simulink model "Galvo_sys_Ccont_Pcont_cc_nosub_bandwidth_v69_linmod"  (R2015a)
settings: Solver=ode45  StartTime=0.0  StopTime=10.0  RelTol=1e-3
undefined symbols (not defined in the file or in its folder): ccKp, dPosMax, JR, KEL, KEMF, KFR, KSH, KTB, Lc, RL, Rsh
libraries: simulink x2
settings Model: DataDictionary=modelDesignData_Galvo_sys_Ccont_Pcont.sldd  Creator=mainster  LastModifiedBy=mainster
settings DebuggingCC: InitInArrayFormatMsg=none

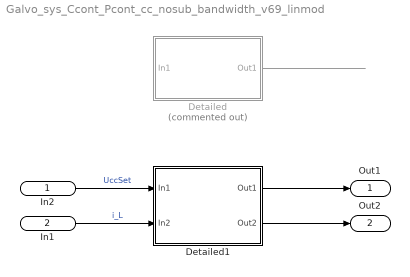
== system Galvo_sys_Ccont_Pcont_cc_nosub_bandwidth_v69_linmod ==
  In2 : Inport
  In1 : Inport  Port=2
  Detailed : Subsystem  Commented=on
  Detailed1 : Subsystem
  Out1 : Outport
  Out2 : Outport  Port=2
  wires:
  ? -> Detailed/1(In1)  "UccSet"
  Detailed/1(Out1) -> ?
  In2/1 -> Detailed1/1(In1)  "UccSet"
  Detailed1/1(Out1) -> Out1/1
  In1/1 -> Detailed1/2(In2)  "i_L"
  Detailed1/2(Out2) -> Out2/1

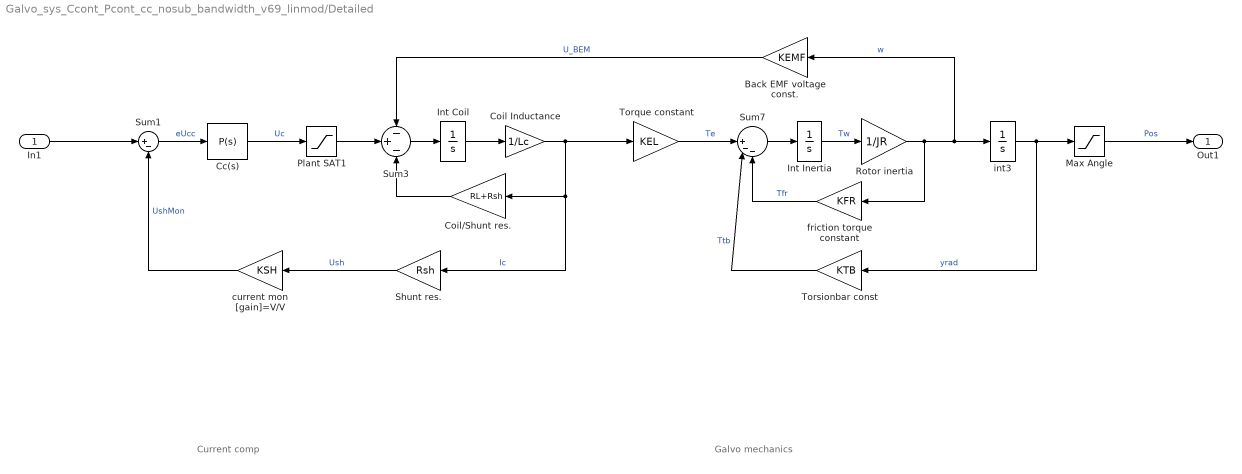
== system Galvo_sys_Ccont_Pcont_cc_nosub_bandwidth_v69_linmod/Detailed ==
  note: Galvo mechanics
  note: Current comp
  In1 : Inport
  Back EMF voltage const. : Gain  RequirementInfo={} %GIDa_1b5a4587_d3eb_4817_81be_45424a09f54c  Gain=KEMF
  Cc(s) : simulink/Continuous/PID Controller  Controller=P  TimeDomain=Continuous-time  SampleTime=-1  IntegratorMethod=Forward Euler  FilterMethod=Forward Euler  Form=Ideal  UseFilter=on  ControllerParametersSource=internal  P=ccKp  I=79241.5509357268  D=0  N=100  InitialConditionSource=internal  InitialConditionForIntegrator=0  InitialConditionForFilter=0  ExternalReset=none  LimitOutput=off  UpperSaturationLimit=inf  LowerSaturationLimit=-inf  LinearizeAsGain=on  AntiWindupMode=none  Kb=1  TrackingMode=off  Kt=1  PParamMin=[]  PParamMax=[]  IParamMin=[]  IParamMax=[]  DParamMin=[]  DParamMax=[]  NParamMin=[]  NParamMax=[]  KbParamMin=[]  KbParamMax=[]  KtParamMin=[]  KtParamMax=[]  POutMin=[]  POutMax=[]  IOutMin=[]  IOutMax=[]  DOutMin=[]  DOutMax=[]  NOutMin=[]  NOutMax=[]  KbOutMin=[]  KbOutMax=[]  KtOutMin=[]  KtOutMax=[]  IntegratorOutMin=[]  IntegratorOutMax=[]  FilterOutMin=[]  FilterOutMax=[]  SumOutMin=[]  SumOutMax=[]  SumI1OutMin=[]  SumI1OutMax=[]  SumI2OutMin=[]  SumI2OutMax=[]  SumI3OutMin=[]  SumI3OutMax=[]  SumDOutMin=[]  SumDOutMax=[]  SaturationOutMin=[]  SaturationOutMax=[]  IntegratorContinuousStateAttributes=''  IntegratorStateMustResolveToSignalObject=off  IntegratorRTWStateStorageClass=Auto  FilterContinuousStateAttributes=''  FilterStateMustResolveToSignalObject=off  FilterRTWStateStorageClass=Auto  DifferentiatorICPrevScaledInput=0  DifferentiatorOutMin=[]  DifferentiatorOutMax=[]
  Coil Inductance : Gain  Gain=1/Lc
  Coil/Shunt res. : Gain  Gain=RL+Rsh
  Int Coil : Integrator
  Int Inertia : Integrator
  Max Angle : Saturate  UpperLimit=0.5*dPosMax  LowerLimit=-0.5*dPosMax
      settings: AttributesFormatString=Max=%<UpperLimit>\nMin=%<LowerLimit>
  Plant SAT1 : Saturate  UpperLimit=30  LowerLimit=-30
      settings: AttributesFormatString=U_lim=+-%<UpperLimit>V
  Rotor inertia : Gain  Gain=1/JR
  Shunt res. : Gain  Gain=Rsh
  Sum1 : Sum  Inputs=|+-
  Sum3 : Sum  Inputs=-+-
  Sum7 : Sum  Inputs=||+--
  Torque constant : Gain  Gain=KEL
  Torsionbar const : Gain  Gain=KTB
  current mon [gain]=V/V : Gain  RequirementInfo={} %GIDa_afd0055d_3b4e_4389_b2ee_a23c394953dc  Gain=KSH
      settings: AttributesFormatString=KSH=%<Gain>
  friction torque constant : Gain  Gain=KFR
  int3 : Integrator
  Out1 : Outport
  wires:
  Int Inertia/1 -> Rotor inertia/1  "Tw"
  Sum7/1 -> Int Inertia/1
  Rotor inertia/1 -> int3/1, Back EMF voltage const./1, friction torque constant/1  "w"
  friction torque constant/1 -> Sum7/3  "Tfr"
  Max Angle/1 -> Out1/1  "Pos"
  Torque constant/1 -> Sum7/1  "Te"
  Torsionbar const/1 -> Sum7/2  "Ttb"
  Coil Inductance/1 -> Shunt res./1, Coil/Shunt res./1, Torque constant/1  "Ic"
  Coil/Shunt res./1 -> Sum3/3
  int3/1 -> Max Angle/1, Torsionbar const/1  "yrad"
  Sum3/1 -> Int Coil/1
  Int Coil/1 -> Coil Inductance/1
  Cc(s)/1 -> Plant SAT1/1  "Uc"
  Shunt res./1 -> current mon [gain]=V/V/1  "Ush"
  current mon [gain]=V/V/1 -> Sum1/2  "UshMon"
  Plant SAT1/1 -> Sum3/2
  Back EMF voltage const./1 -> Sum3/1  "U_BEM"
  Sum1/1 -> Cc(s)/1  "eUcc"
  In1/1 -> Sum1/1

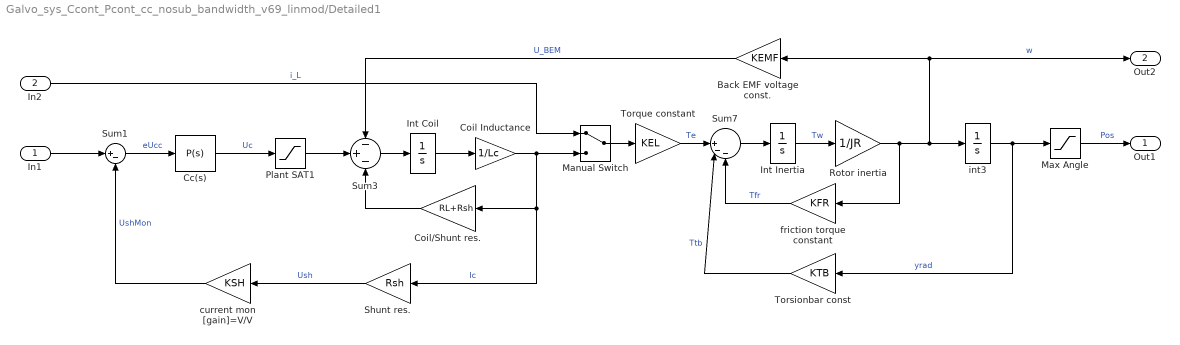
== system Galvo_sys_Ccont_Pcont_cc_nosub_bandwidth_v69_linmod/Detailed1 ==
  In1 : Inport
  In2 : Inport  Port=2
  Back EMF voltage const. : Gain  RequirementInfo={} %GIDa_2b4a7570_bc29_44df_a986_5abe18d0e538  Gain=KEMF
  Cc(s) : simulink/Continuous/PID Controller  Controller=P  TimeDomain=Continuous-time  SampleTime=-1  IntegratorMethod=Forward Euler  FilterMethod=Forward Euler  Form=Ideal  UseFilter=on  ControllerParametersSource=internal  P=ccKp  I=79241.5509357268  D=0  N=100  InitialConditionSource=internal  InitialConditionForIntegrator=0  InitialConditionForFilter=0  ExternalReset=none  LimitOutput=off  UpperSaturationLimit=inf  LowerSaturationLimit=-inf  LinearizeAsGain=on  AntiWindupMode=none  Kb=1  TrackingMode=off  Kt=1  PParamMin=[]  PParamMax=[]  IParamMin=[]  IParamMax=[]  DParamMin=[]  DParamMax=[]  NParamMin=[]  NParamMax=[]  KbParamMin=[]  KbParamMax=[]  KtParamMin=[]  KtParamMax=[]  POutMin=[]  POutMax=[]  IOutMin=[]  IOutMax=[]  DOutMin=[]  DOutMax=[]  NOutMin=[]  NOutMax=[]  KbOutMin=[]  KbOutMax=[]  KtOutMin=[]  KtOutMax=[]  IntegratorOutMin=[]  IntegratorOutMax=[]  FilterOutMin=[]  FilterOutMax=[]  SumOutMin=[]  SumOutMax=[]  SumI1OutMin=[]  SumI1OutMax=[]  SumI2OutMin=[]  SumI2OutMax=[]  SumI3OutMin=[]  SumI3OutMax=[]  SumDOutMin=[]  SumDOutMax=[]  SaturationOutMin=[]  SaturationOutMax=[]  IntegratorContinuousStateAttributes=''  IntegratorStateMustResolveToSignalObject=off  IntegratorRTWStateStorageClass=Auto  FilterContinuousStateAttributes=''  FilterStateMustResolveToSignalObject=off  FilterRTWStateStorageClass=Auto  DifferentiatorICPrevScaledInput=0  DifferentiatorOutMin=[]  DifferentiatorOutMax=[]
  Coil Inductance : Gain  Gain=1/Lc
  Coil/Shunt res. : Gain  Gain=RL+Rsh
  Int Coil : Integrator
  Int Inertia : Integrator
  Manual Switch : ManualSwitch
  Max Angle : Saturate  UpperLimit=0.5*dPosMax  LowerLimit=-0.5*dPosMax
      settings: AttributesFormatString=Max=%<UpperLimit>\nMin=%<LowerLimit>
  Plant SAT1 : Saturate  UpperLimit=30  LowerLimit=-30
      settings: AttributesFormatString=U_lim=+-%<UpperLimit>V
  Rotor inertia : Gain  Gain=1/JR
  Shunt res. : Gain  Gain=Rsh
  Sum1 : Sum  Inputs=|+-
  Sum3 : Sum  Inputs=-+-
  Sum7 : Sum  Inputs=||+--
  Torque constant : Gain  Gain=KEL
  Torsionbar const : Gain  Gain=KTB
  current mon [gain]=V/V : Gain  RequirementInfo={} %GIDa_22274a97_2114_4aad_a4b8_b60c8b944f37  Gain=KSH
      settings: AttributesFormatString=KSH=%<Gain>
  friction torque constant : Gain  Gain=KFR
  int3 : Integrator
  Out1 : Outport
  Out2 : Outport  Port=2
  wires:
  Int Inertia/1 -> Rotor inertia/1  "Tw"
  Sum7/1 -> Int Inertia/1
  Rotor inertia/1 -> int3/1, Out2/1, Back EMF voltage const./1, friction torque constant/1  "w"
  friction torque constant/1 -> Sum7/3  "Tfr"
  Max Angle/1 -> Out1/1  "Pos"
  Torque constant/1 -> Sum7/1  "Te"
  Torsionbar const/1 -> Sum7/2  "Ttb"
  Coil Inductance/1 -> Shunt res./1, Coil/Shunt res./1, Manual Switch/2  "Ic"
  Coil/Shunt res./1 -> Sum3/3
  int3/1 -> Max Angle/1, Torsionbar const/1  "yrad"
  Sum3/1 -> Int Coil/1
  Int Coil/1 -> Coil Inductance/1
  Cc(s)/1 -> Plant SAT1/1  "Uc"
  Shunt res./1 -> current mon [gain]=V/V/1  "Ush"
  current mon [gain]=V/V/1 -> Sum1/2  "UshMon"
  Plant SAT1/1 -> Sum3/2
  Back EMF voltage const./1 -> Sum3/1  "U_BEM"
  Sum1/1 -> Cc(s)/1  "eUcc"
  In1/1 -> Sum1/1
  In2/1 -> Manual Switch/1  "i_L"
  Manual Switch/1 -> Torque constant/1
